simulink model "s0221c"  (Simulink 6.0)
settings: Solver=ode3  SolverMode=SingleTasking  StartTime=0.0  StopTime=900  FixedStep=1  MaxStep=1  RelTol=1e-3  AbsTol=1e-6
values from neighbouring files (symbols this model uses):
  DAdach = DAdachVec(i)    [m0221d.m]    (also in m0224.m = 0)
  Dudach = 0    [m0221d.m]    (also in m0224.m = DudachVec(i))
settings Model: LastModifiedBy=Froriep
settings DataIOCC: LimitDataPoints=off  SaveOutput=off  SaveTime=off
settings OptimizationCC: BooleanDataType=off
settings DebuggingCC: SolverPrmCheckMsg=none
settings HardwareCC: TargetUnknown=on
settings GRTTargetCC: ModelReferenceCompliant=off  MatFileLogging=off

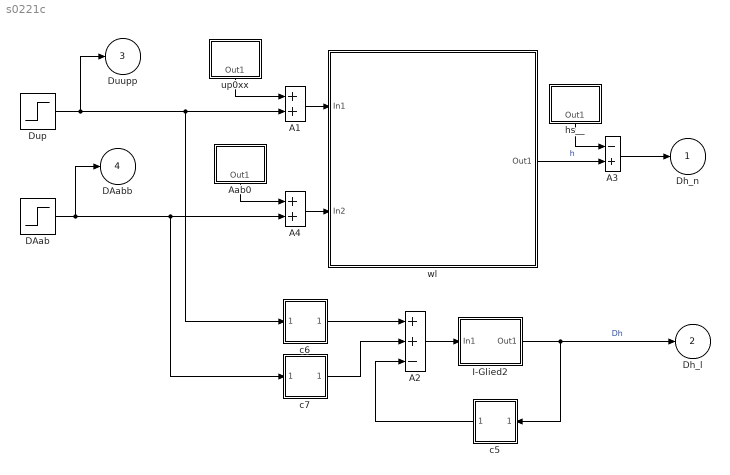
== system s0221c ==
  A1 : Sum  SaturateOnIntegerOverflow=on  InputSameDT=on
  A2 : Sum  Inputs=++-  SaturateOnIntegerOverflow=on  InputSameDT=on
  A3 : Sum  Inputs=-+  SaturateOnIntegerOverflow=on  InputSameDT=on
  A4 : Sum  SaturateOnIntegerOverflow=on  InputSameDT=on
  Aab0 : Subsystem  Orientation=down  mask(Konstante){@1=Aab0}
      mask prompts: @1 "Wert"
      mask help: Konstante
      mask init:
      | Konst=@1;
      mask Display: disp('Aab0')
  DAab : Step  Time=50  After=DAdach  SampleTime=0
  Dup : Step  Time=50  After=Dudach  SampleTime=0
  I-Glied2 : Subsystem  mask(I-Glied){@1=0}
      mask prompts: @1 "Anfangswert"
      mask help: I-Glied
      mask init:
      | x0=@1;
      mask Display: disp('I-Glied')
  c5 : Subsystem  Orientation=left  mask(P-Glied){@1=a0}
      mask prompts: @1 "Beiwert"
      mask help: P-Glied
      mask init:
      | Kp=@1;
      mask Display: disp('a0')
  c6 : Subsystem  mask(P-Glied){@1=b01}
      mask prompts: @1 "Beiwert"
      mask help: P-Glied
      mask init:
      | Kp=@1;
      mask Display: disp('b01')
  c7 : Subsystem  mask(P-Glied){@1=b02}
      mask prompts: @1 "Beiwert"
      mask help: P-Glied
      mask init:
      | Kp=@1;
      mask Display: disp('b02')
  hs__ : Subsystem  Orientation=down  mask(Konstante){@1=hs}
      mask prompts: @1 "Wert"
      mask help: Konstante
      mask init:
      | Konst=@1;
      mask Display: disp('hs')
  up0xx : Subsystem  Orientation=down  mask(Konstante){@1=up0}
      mask prompts: @1 "Wert"
      mask help: Konstante
      mask init:
      | Konst=@1;
      mask Display: disp('up0')
  wl : Subsystem
      mask Display: disp('Nichtlineares\nFüllstandsmodell')
  Dh_n : Outport
  Dh_l : Outport  Port=2
  Duupp : Outport  Port=3
  DAabb : Outport  Port=4
  wires:
  Aab0/1(Out1) -> A4/1
  up0xx/1(Out1) -> A1/1
  hs__/1(Out1) -> A3/1
  A3/1 -> Dh_n/1
  A1/1 -> wl/1(In1)
  A4/1 -> wl/2(In2)
  A2/1 -> I-Glied2/1(In1)
  c5/1(Out1) -> A2/3
  c6/1(Out1) -> A2/1
  c7/1(Out1) -> A2/2
  I-Glied2/1(Out1) -> Dh_l/1, c5/1(In1)  "Dh"
  Dup/1 -> A1/2, c6/1(In1), Duupp/1
  DAab/1 -> A4/2, c7/1(In1), DAabb/1
  wl/1(Out1) -> A3/2  "h"

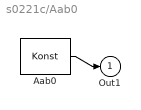
== system s0221c/Aab0 ==
  Aab0 : Constant  Value=Konst
  Out1 : Outport
  wires:
  Aab0/1 -> Out1/1

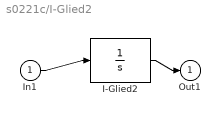
== system s0221c/I-Glied2 ==
  In1 : Inport  Port=1  LatchInput=off
  I-Glied2 : Integrator  InitialCondition=x0
  Out1 : Outport
  wires:
  In1/1 -> I-Glied2/1
  I-Glied2/1 -> Out1/1

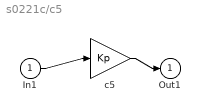
== system s0221c/c5 ==
  In1 : Inport  Port=1  LatchInput=off
  c5 : Gain  Gain=Kp  SaturateOnIntegerOverflow=on
  Out1 : Outport
  wires:
  In1/1 -> c5/1
  c5/1 -> Out1/1

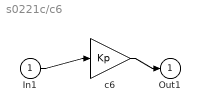
== system s0221c/c6 ==
  In1 : Inport  Port=1  LatchInput=off
  c6 : Gain  Gain=Kp  SaturateOnIntegerOverflow=on
  Out1 : Outport
  wires:
  In1/1 -> c6/1
  c6/1 -> Out1/1

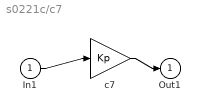
== system s0221c/c7 ==
  In1 : Inport  Port=1  LatchInput=off
  c7 : Gain  Gain=Kp  SaturateOnIntegerOverflow=on
  Out1 : Outport
  wires:
  In1/1 -> c7/1
  c7/1 -> Out1/1

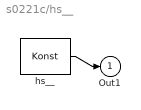
== system s0221c/hs__ ==
  hs__ : Constant  Value=Konst
  Out1 : Outport
  wires:
  hs__/1 -> Out1/1

== system s0221c/up0xx ==
  up0xx : Constant  Value=Konst
  Out1 : Outport
  wires:
  up0xx/1 -> Out1/1

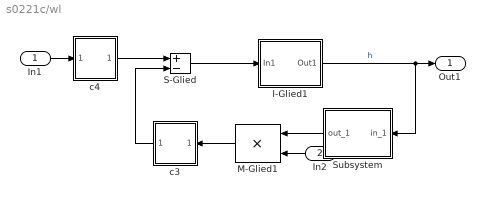
== system s0221c/wl ==
  In1 : Inport  Port=1  LatchInput=off
  In2 : Inport  Orientation=left  Port=2  LatchInput=off
  I-Glied1 : Subsystem  mask(I-Glied){@1=0}
      mask prompts: @1 "Anfangswert"
      mask help: I-Glied
      mask init:
      | x0=@1;
      mask Display: disp('I-Glied')
  M-Glied1 : Product  Orientation=left  SaturateOnIntegerOverflow=on  RndMeth=Zero  InputSameDT=on
  S-Glied : Sum  Inputs=+-  SaturateOnIntegerOverflow=on  InputSameDT=on
  Subsystem : Subsystem  Orientation=left
      mask Display: disp('Wurzel')
  c3 : Subsystem  Orientation=left  mask(P-Glied){@1=c1}
      mask prompts: @1 "Beiwert"
      mask help: P-Glied
      mask init:
      | Kp=@1;
      mask Display: disp('c1')
  c4 : Subsystem  mask(P-Glied){@1=c2}
      mask prompts: @1 "Beiwert"
      mask help: P-Glied
      mask init:
      | Kp=@1;
      mask Display: disp('c2')
  Out1 : Outport
  wires:
  I-Glied1/1(Out1) -> Subsystem/1(in_1), Out1/1  "h"
  c3/1(Out1) -> S-Glied/2
  Subsystem/1(out_1) -> M-Glied1/1
  M-Glied1/1 -> c3/1(In1)
  S-Glied/1 -> I-Glied1/1(In1)
  c4/1(Out1) -> S-Glied/1
  In1/1 -> c4/1(In1)
  In2/1 -> M-Glied1/2

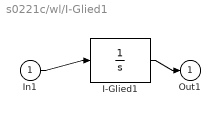
== system s0221c/wl/I-Glied1 ==
  In1 : Inport  Port=1  LatchInput=off
  I-Glied1 : Integrator  InitialCondition=x0
  Out1 : Outport
  wires:
  In1/1 -> I-Glied1/1
  I-Glied1/1 -> Out1/1

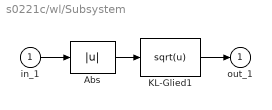
== system s0221c/wl/Subsystem ==
  in_1 : Inport  Port=1  LatchInput=off
  Abs : Abs  SaturateOnIntegerOverflow=on
  KL-Glied1 : Fcn  Expr=sqrt(u)
  out_1 : Outport
  wires:
  KL-Glied1/1 -> out_1/1
  in_1/1 -> Abs/1
  Abs/1 -> KL-Glied1/1

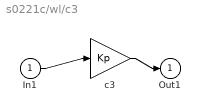
== system s0221c/wl/c3 ==
  In1 : Inport  Port=1  LatchInput=off
  c3 : Gain  Gain=Kp  SaturateOnIntegerOverflow=on
  Out1 : Outport
  wires:
  In1/1 -> c3/1
  c3/1 -> Out1/1

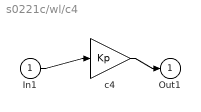
== system s0221c/wl/c4 ==
  In1 : Inport  Port=1  LatchInput=off
  c4 : Gain  Gain=Kp  SaturateOnIntegerOverflow=on
  Out1 : Outport
  wires:
  In1/1 -> c4/1
  c4/1 -> Out1/1
